simulink model "Blink_Led"  (R2022b)
settings: Solver=VariableStepDiscrete  StartTime=0.0  StopTime=10.0  MaxStep=0.1  RelTol=1e-3
settings Model: Creator=yasso  LastModifiedBy=yasso

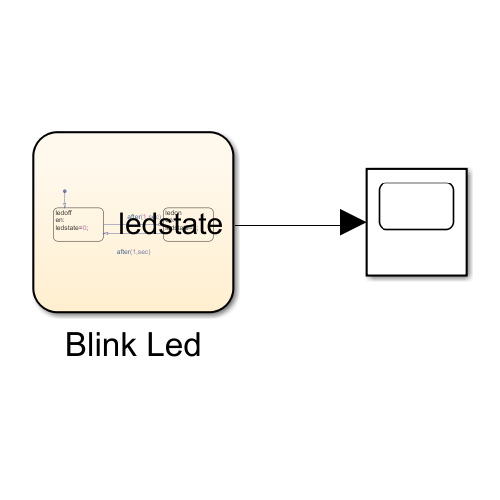
[thumbnail: Simulink's stored preview of the top-level diagram]
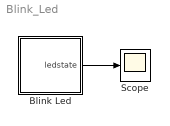
== system Blink_Led ==
  Blink Led : Stateflow chart  TreatAsAtomicUnit=on
  Scope : Scope
  wires:
  Blink Led/1(ledstate) -> Scope/1

== stateflow chart Blink_Led/Blink Led ==
  state ledoff
    en:
    ledstate=0;
  state ledon
    en:
    ledstate=1;
  (default) -> ledoff
  ledoff -> ledon : after(1,sec)
  ledon -> ledoff : after(1,sec)
  data: ledstate output double
